simulink model "SOSF_FLL"  (R2024b)
settings: Solver=VariableStepAuto  StartTime=0.0  StopTime=1  RelTol=1e-3
undefined symbols (not defined in the file or in its folder): magnitude
libraries: spsabctoAlphaBetaZeroLib x1
settings Model: Creator=Anikait  LastModifiedBy=kaush
settings RTWCC: GPUComputeCapability=3.5

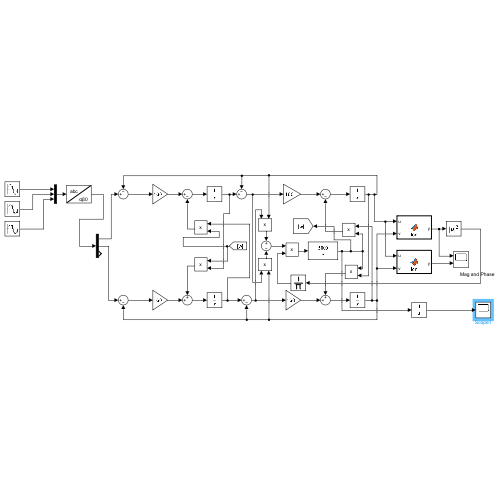
[thumbnail: Simulink's stored preview of the top-level diagram]
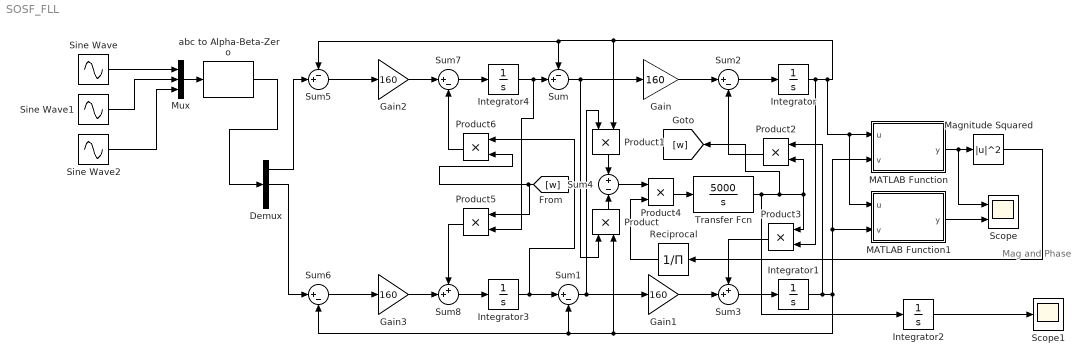
== system SOSF_FLL ==
  note: Mag and Phase
  Demux : Demux  Outputs=3
  Gain{,1..3} (4 alike) : Gain  Gain=160
  Integrator{,1..4} (5 alike) : Integrator  InitialCondition=1
  MATLAB Function : MATLAB Function  TreatAsAtomicUnit=on
  MATLAB Function1 : MATLAB Function  TreatAsAtomicUnit=on
  Magnitude Squared : Math  Operator=magnitude^2
  Mux : Mux  Inputs=3
  Product{,1..6} (7 alike) : Product
  Reciprocal : Product  Inputs=/  RndMeth=Zero  SaturateOnIntegerOverflow=on
  Scope : Scope  NumInputPorts=2
  Scope1 : Scope
  Sine Wave : Sin  Amplitude=311  Frequency=2*pi*50  SampleTime=1/10000
  Sine Wave1 : Sin  Amplitude=311  Frequency=2*pi*50  Phase=2*pi/3  SampleTime=1/10000
  Sine Wave2 : Sin  Amplitude=311  Frequency=2*pi*50  Phase=4*pi/3  SampleTime=1/10000
  Sum : Sum  Inputs=-+|
  Sum{1..2,6..7} (4 alike) : Sum  Inputs=|+-
  Sum3 : Sum  Inputs=++|
  Sum4 : Sum  Inputs=+-
  Sum5 : Sum  Inputs=-+|
  Sum8 : Sum  Inputs=++|
  Transfer Fcn : TransferFcn  Numerator=[5000]  Denominator=[1 0]
  abc to Alpha-Beta-Zero : spsabctoAlphaBetaZeroLib/abc to Alpha-Beta-Zero
  wires:
  Integrator2/1 -> Scope1/1
  Sum2/1 -> Integrator/1
  Product3/1 -> Sum3/1
  abc to Alpha-Beta-Zero/1 -> Demux/1
  Magnitude Squared/1 -> Reciprocal/1
  Sum4/1 -> Product4/1
  Product1/1 -> Sum4/1
  MATLAB Function1/1(y) -> Scope/2
  MATLAB Function/1(y) -> Scope/1, Magnitude Squared/1
  Transfer Fcn/1 -> [w], Product3/1, Product2/2, Integrator2/1
  Product4/1 -> Transfer Fcn/1
  Product/1 -> Sum4/2
  Gain/1 -> Sum2/1
  Product2/1 -> Sum2/2
  Mux/1 -> abc to Alpha-Beta-Zero/1
  Sine Wave2/1 -> Mux/3
  Gain1/1 -> Sum3/2
  Sum/1 -> Product/1, Gain/1
  Sum1/1 -> Product1/1, Gain1/1
  Sine Wave/1 -> Mux/1
  Sine Wave1/1 -> Mux/2
  Integrator/1 -> Product3/2, MATLAB Function1/1(u), MATLAB Function/1(u), Product1/2, Sum5/1, Sum/1
  Reciprocal/1 -> Product4/2
  Integrator1/1 -> Product2/1, MATLAB Function1/2(v), MATLAB Function/2(v), Product/2, Sum6/2, Sum1/2
  Sum3/1 -> Integrator1/1
  Sum5/1 -> Gain2/1
  Sum6/1 -> Gain3/1
  Gain2/1 -> Sum7/1
  Gain3/1 -> Sum8/2
  Sum8/1 -> Integrator3/1
  Sum7/1 -> Integrator4/1
  Integrator3/1 -> Product6/1, Sum1/1
  [w] -> Product6/2, Product5/1
  Integrator4/1 -> Product5/2, Sum/2
  Product6/1 -> Sum7/2
  Product5/1 -> Sum8/1
  Demux/1 -> Sum5/2
  Demux/2 -> Sum6/1

== matlab function SOSF_FLL/MATLAB Function ==
  data: u input; y output; v input
function y = fcn(u,v)

y = sqrt((u^2)+(v^2));

== matlab function SOSF_FLL/MATLAB Function1 ==
  data: u input; y output; v input
function y = fcn(u,v)

y = atan(v/u);
